simulink model "test_simulink"  (R2024b)
settings: Solver=ode45  StartTime=0.0  StopTime=100  RelTol=1e-3
undefined symbols (not defined in the file or in its folder): experiment, veh
libraries: simulink x1, simulink_extras x1, autolibshared x1
settings Model: Creator=caugu  LastModifiedBy=caugu

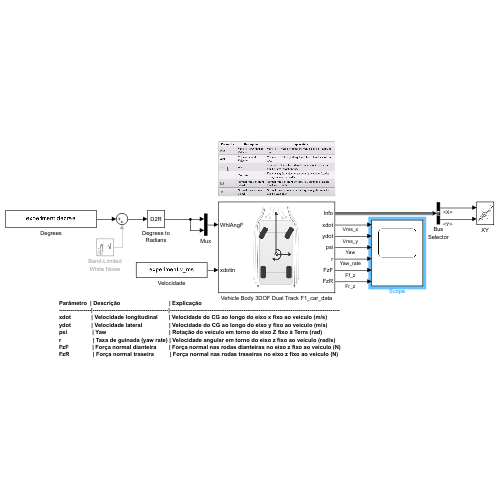
[thumbnail: Simulink's stored preview of the top-level diagram]
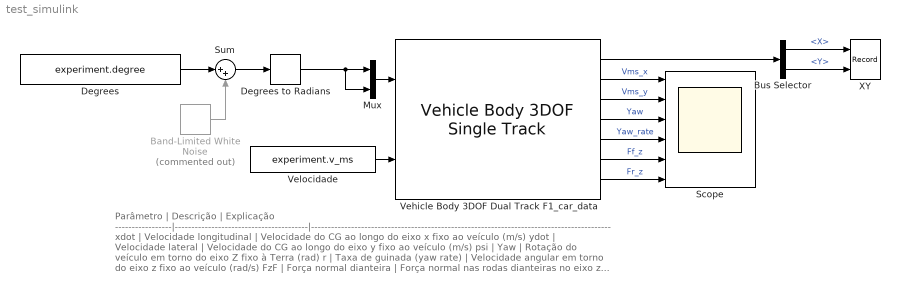
== system test_simulink ==
  note: Parâmetro | Descrição | Explicação
      | -----------------|----------------------------------------|------------------------------------------------------------------------------------------
      | xdot | Velocidade longitudinal | Velocidade do CG ao longo do eixo x fixo ao veículo (m/s)
      | ydot | Velocidade lateral | Velocidade do CG ao longo do eixo y fixo ao veículo (m/s)
      | psi | Yaw | Rotação do veículo em torno do eixo Z fixo à Terra (rad)
      | r | Taxa de guinada (yaw rate) | Velocidade angular em torno do eixo z fixo ao veículo (rad/s)
      | FzF | Força normal dianteira | Força normal nas rodas dianteiras no eixo z fixo ao veículo (N)
      | FzR | Força normal traseira | Força normal nas rodas traseiras no eixo z fixo ao veículo (N)
  Band-Limited White Noise : simulink/Sources/Band-Limited White Noise  Commented=on  Cov=[0.2]  Ts=0.1  seed=[23341]
  Bus Selector : BusSelector  OutputSignals=InertFrm.Cg.Disp.X,InertFrm.Cg.Disp.Y
  Degrees : Constant  Value=experiment.degree
  Degrees to Radians : simulink_extras/Transformations/Degrees to Radians
  Mux : Mux  Inputs=2
  Scope : Scope  NumInputPorts=6
  Sum : Sum  Inputs=|++
  Vehicle Body 3DOF Dual Track F1_car_data : autolibshared/Vehicle Body 3DOF Single Track  trackMode=Dual  inputMode=External longitudinal velocity  frontSteerMode=on  rearSteerMode=off  windMode=off  muMode=off  extFMode=off  extMMode=off  htchFMode=off  htchMMode=off  extXo=off  extpsio=off  extxdoto=off  extro=off  extYo=off  extTamb=off  extydoto=off  aMode=2  NF=2  NR=2  m=veh.massa_total_kg  a=veh.dist_cg_eixo_dianteiro_m  b=veh.dist_cg_eixo_traseiro_m  h=veh.altura_cg_m  dh=1  hh=0.2  X_o=0  xdot_o=0  CalphaMode=off  sigmaMode=on  d=0  hl=0  w=[1.4,1.4]  Cy_f=12e3  Cy_r=11e3  sigma_f=.1  sigma_r=.1  alpha_f_brk=[-.1 .1]  Cy_f_data=[-9e3 9e3]  alpha_r_brk=[-.1 .1]  Cy_r_data=[-9e3 9e3]  Y_o=0  ydot_o=0  Izz=4000  psi_o=0  r_o=0  Af=veh.area_frontal_m2  Cd=veh.coef_arrasto_cd  Cl=veh.coef_sutentacao_cl  Cpm=.1  beta_w=[0 0.01:0.01:0.3]  Cs=[0:0.03:0.9]  Cym=[0 1e-6:0.01:0.3]  Pabs=101325  Tair=273+25  g=9.81  mu=1  xdot_tol=.01  Fznom=5000  Fxtire_sat=7e4  Fytire_sat=7e4  longOff=0  latOff=0  vertOff=0  wrapAng=off
      settings: LibrarySourceBlock=vehdynlibeom/Vehicle Body 3DOF Dual Track
  Velocidade : Constant  Value=experiment.v_ms
  XY : Record  FileSettingsInternal="{\"entries\":[{\"content\":{\"excelSettings\":{\"content\":{},\"type\":\"Streamout.ExcelSettings\"}},\"type\":\"Streamout.FileSettingStorage\",\"uuid\":\"\"}],\"packageUris\":[\"http:\\/\\/schema.mathworks.com\\/mf0\\/streamout_blocks\\/R2020a\"],\"version\":\"1.0\"}"  Layout=[1 1]  SignalsInternal="{\"entries\":[{\"content\":{\"signals\":[{\"content\":{\"blockPath\":[],\"dimensions\":[1],\"domain\":\"\",\"lineColor\":\"#a2142f\",\"plots\":[ 1 ],\"port\":1,\"sid\":[\"\"],\"signalID\":1,\"signalName\":\"<X>\"},\"type\":\"RecordBlkView.Signal\",\"uuid\":\"\"},{\"content\":{\"blockPath\":[],\"dimensions\":[1],\"domain\":\"\",\"lineColor\":\"#139fff\",\"plots\":[ 1 ],\"port\":2,\"sid\":[\"\"],\"signalID\":2,\"signalName\":\"<Y>\"},\"type\":\"RecordBlkView.Signal\",\"uuid\":\"\"}]},\"type\":\"RecordBlkView.InputSignals\",\"uuid\":\"\"}],\"packageUris\":[\"http:\\/\\/schema.mathworks.com\\/mf0\\/streamout_blocks\\/R2020a\"],\"version\":\"1.0\"}"  VisualizationBindings="{\"xyplotplugin\":{\"info\":[{\"series\":[{\"bindingParametersList\":[{\"parameter\":\"X-Axis\",\"signalID\":1,\"signalName\":\"<X>\"},{\"parameter\":\"Y-Axis\",\"signalID\":2,\"signalName\":\"<Y>\"}],\"seriesID\":0}],\"subplotID\":1}]}}"  CompatibilityTag=XY  st=-1
  wires:
  Degrees to Radians/1 -> Mux/2, Mux/1
  Vehicle Body 3DOF Dual Track F1_car_data/2 -> Scope/1  "Vms_x"
  Vehicle Body 3DOF Dual Track F1_car_data/3 -> Scope/2  "Vms_y"
  Vehicle Body 3DOF Dual Track F1_car_data/4 -> Scope/3  "Yaw"
  Vehicle Body 3DOF Dual Track F1_car_data/5 -> Scope/4  "Yaw_rate"
  Vehicle Body 3DOF Dual Track F1_car_data/6 -> Scope/5  "Ff_z"
  Vehicle Body 3DOF Dual Track F1_car_data/7 -> Scope/6  "Fr_z"
  Velocidade/1 -> Vehicle Body 3DOF Dual Track F1_car_data/2
  Vehicle Body 3DOF Dual Track F1_car_data/1 -> Bus Selector/1
  Bus Selector/2 -> XY/2  "<Y>"
  Bus Selector/1 -> XY/1  "<X>"
  Mux/1 -> Vehicle Body 3DOF Dual Track F1_car_data/1
  Degrees/1 -> Sum/1
  Sum/1 -> Degrees to Radians/1
  Band-Limited White Noise/1 -> Sum/2
